simulink model "UrbanCHIL"  (Simulink 8.1)
settings: Solver=ode1  StartTime=0.0  StopTime=inf  FixedStep=Ts  MaxStep=1e-3  RelTol=1e-3
PostLoadFcn:
  | NREL_Mode=1; BANSHEE_init;
InitFcn:
  | NREL_Mode=1; BANSHEE_init;
values from neighbouring files (symbols this model uses):
  DER_REL = xlsread('DER_relay.xlsx')    [relay_settings_init.m]
  F0 = xlsread('F0_relay_banshee.xlsx')    [relay_settings_init.m]
  F2 = xlsread('F2_relay_banshee.xlsx')    [relay_settings_init.m]
  F3 = xlsread('F3_relay_banshee.xlsx')    [relay_settings_init.m]
  F4 = xlsread('F4_relay_nrel.xlsx')    [relay_settings_init.m]
  Ts = 100E-6    (= 0.0001)    [BANSHEE_init.m]    (also in Ghost_init.m)
undefined symbols (not defined in the file or in its folder): CBID, communications_lib, Feeder2_lib, Feeder3_lib, Feeder4_lib, generic_ethernet_cb, Left, relay_housing_lib, SM_UtilityService, SS_COMMUNICATION, SS_F2_RELAY_HOUSING, SS_F3_RELAY_HOUSING, SS_Feeder2, SS_Feeder3, SS_Feeder4, Stim, type, utility_service_lib, V
libraries: simulink x80, relay_modbus_lib x80, breaker_lib x46, rtio_generic_modbus x45, cables_lib x30, rtlab x22, Load_lib x21, powerlib x20, transformer_lib x19, ssn_lib x13, artemis x6, BESS_lib x4
(part 3 of 6)

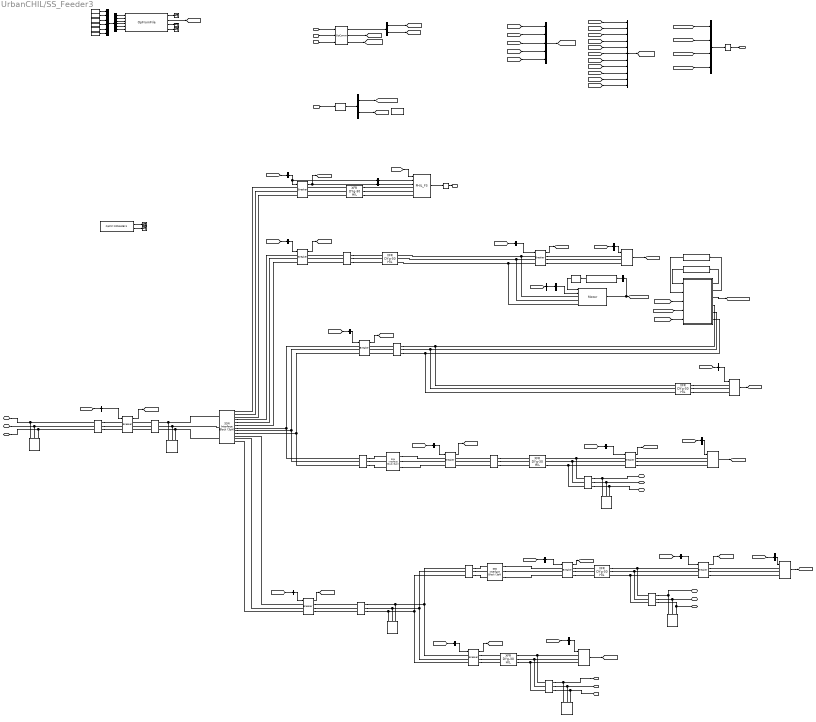
== system UrbanCHIL/SS_Feeder3 ==
  note: Signal for this Cb will come from a SEL relay
  note: connect to F2
  note: connect to F2
  note: connect to F2
  note: % Copyright (c) 2016 Massachusetts Institute of Technology
      | % Permission is hereby granted, free of charge, to any person obtaining a copy of this
      | % software and associated documentation files (the "Software"), to deal in the Software
      | % without restriction, including without limitation the rights to use, copy, modify,
      | % merge, publish, distribute, sublicense, and/or sell copies of the Software, and to
      | % permit persons to whom the Software is furnished to do so, subject to the following
      | % conditions:
      | %
      | %
      | % The above copyright notice and this permission notice shall be included in
      | % all copies or substantial portions of the Software.
      | %
      | % THE SOFTWARE IS PROVIDED "AS IS", WITHOUT WARRANTY OF ANY KIND, EXPRESS OR IMPLIED,
      | % INCLUDING BUT NOT LIMITED TO THE WARRANTIES OF MERCHANTABILITY, FITNESS FOR A
      | % PARTICULAR PURPOSE AND NONINFRINGEMENT. IN NO EVENT SHALL THE AUTHORS OR COPYRIGHT
      | % HOLDERS BE LIABLE FOR ANY CLAIM, DAMAGES OR OTHER LIABILITY, WHETHER IN AN ACTION
      | % OF CONTRACT, TORT OR OTHERWISE, ARISING FROM, OUT OF OR IN CONNECTION WITH THE
      | % SOFTWARE OR THE USE OR OTHER DEALINGS IN THE SOFTWARE.
      | %
      | %
      | %%
  note: PHIL interface
  RELAY_IN : Inport
  LOAD_IN : Inport  Port=2
  SC_CMD : Inport  Port=3
  PHIL_I : Inport  Port=4
  1000 kVA : transformer_lib/XFR DYg-30 HIL  Rating=1000  Vp=13800  Vs=480  Z=5.56  XR=5.49
  1000 kVA1 : transformer_lib/XFR DYg-30 HIL  Rating=1000  Vp=13800  Vs=480  Z=5.56  XR=5.49
  200 HP chiller compressor : Load_lib/200 HP chiller compressor
  2000 kVA : transformer_lib/XFR DYg-30 HIL  Rating=2000  Vp=13800  Vs=480  Z=5.75  XR=5.7
  2000 kVA1 : transformer_lib/XFR DYg-30 HIL  Rating=2000  Vp=13800  Vs=480  Z=5.75  XR=5.7
  2500 kVA : transformer_lib/XFR DYg-30 HIL  Rating=2500  Vp=13800  Vs=480  Z=5.75  XR=6.6
  2500 kVA1 : transformer_lib/XFR DYg-30 HIL  Rating=5000  Vp=13800  Vs=4160  Z=5.75  XR=6.6
  448 kvar inductor at 13.8kV  to cancel kvar produced by the stublines1 : powerlib/Elements/Three-Phase Parallel RLC Load  LConnTagsString=A|B|C  Configuration=Y (grounded)  NominalVoltage=13800  NominalFrequency=60  ActivePower=10e3  InductivePower=448e3  CapacitivePower=0  Measurements=None  LoadType=constant Z
  500kcmil-Mutual1 : cables_lib/500kcmil-Mutual  length=10  par_sets=1  ratio=3
  500kcmil-Mutual2 : cables_lib/500kcmil-Mutual  length=10  par_sets=1  ratio=3
  500kcmil-Mutual3 : cables_lib/500kcmil-Mutual  length=100  par_sets=1  ratio=3
  500kcmil-Mutual4 : cables_lib/500kcmil-Mutual  length=10  par_sets=1  ratio=3
  500kcmil-Mutual5 : cables_lib/500kcmil-Mutual  length=1000  par_sets=1  ratio=3
  6 kvar inductor at 480V  to cancel kvar produced by the stublines1 : powerlib/Elements/Three-Phase Parallel RLC Load  LConnTagsString=A|B|C  Configuration=Y (grounded)  NominalVoltage=480  NominalFrequency=60  ActivePower=1e3  InductivePower=6e3  CapacitivePower=0  Measurements=None  LoadType=constant Z
  6 kvar inductor at 480V  to cancel kvar produced by the stublines2 : powerlib/Elements/Three-Phase Parallel RLC Load  LConnTagsString=A|B|C  Configuration=Y (grounded)  NominalVoltage=480  NominalFrequency=60  ActivePower=1e3  InductivePower=6e3  CapacitivePower=0  Measurements=None  LoadType=constant Z
  6 kvar inductor at 480V  to cancel kvar produced by the stublines3 : powerlib/Elements/Three-Phase Parallel RLC Load  LConnTagsString=A|B|C  Configuration=Y (grounded)  NominalVoltage=480  NominalFrequency=60  ActivePower=0  InductivePower=6e3  CapacitivePower=0  Measurements=None  LoadType=constant Z
  Bus Creator2 : BusCreator
  Bus Creator3 : BusCreator  Inputs=5
  Bus Creator5 : BusCreator  Inputs=11
  Bus Selector : BusSelector  OutputSignals=motor
  Bus Selector1 : BusSelector  OutputSignals=F3_CB_4
  Bus Selector10 : BusSelector  OutputSignals=F3_CB_5
  Bus Selector11 : BusSelector  OutputSignals=P6
  Bus Selector12 : BusSelector  OutputSignals=F3_CB_9
  Bus Selector13 : BusSelector  OutputSignals=F3_CB_3
  Bus Selector14 : BusSelector  OutputSignals=F3_CB_8
  Bus Selector15 : BusSelector  OutputSignals=CHP_cmds,IO_scaling
  Bus Selector16 : BusSelector  OutputSignals=Status
  Bus Selector17 : BusSelector  OutputSignals=RPM
  Bus Selector18 : BusSelector  OutputSignals=LoadProfile,TestSeq
  Bus Selector19 : BusSelector  OutputSignals=Logic_trip
  Bus Selector2 : BusSelector  OutputSignals=C6
  Bus Selector20 : BusSelector  OutputSignals=ena2
  Bus Selector21 : BusSelector  OutputSignals=F3_PCC
  Bus Selector22 : BusSelector  OutputSignals=F3_CB_10
  Bus Selector3 : BusSelector  OutputSignals=P4
  Bus Selector4 : BusSelector  OutputSignals=I6
  Bus Selector5 : BusSelector  OutputSignals=C5
  Bus Selector6 : BusSelector  OutputSignals=F3_CB_2
  Bus Selector7 : BusSelector  OutputSignals=F3_CB_7
  Bus Selector8 : BusSelector  OutputSignals=F3_CB_6
  Bus Selector9 : BusSelector  OutputSignals=F3_CB_1
  C1 : cables_lib/500kcmil-Mutual  length=10  par_sets=1  ratio=3
  C2 : cables_lib/500kcmil-Mutual  length=10  par_sets=1  ratio=3
  C301 : cables_lib/500kcmil-Mutual  length=2500  par_sets=1  ratio=3
  C302 : cables_lib/4//0AWG-Mutual  length=2000  par_sets=1  ratio=3
  C303 : cables_lib/500kcmil-Mutual  length=2000  par_sets=1  ratio=3
  C304 : cables_lib/4//0AWG-Mutual  length=1500  par_sets=2  ratio=3
  CHP_Modbus : rtio_generic_modbus/Modbus device  conf_name=CHP_modbus.opal  conf_name_mask=CHP_modbus.xls  sample_time=Ts
  Critical_5 : Load_lib/Dynamic_Load  V=480  kVA=1000  PF=0.9  Ts=Ts
  Critical_6 : Load_lib/Dynamic_Load  V=480  kVA=800  PF=0.9  Ts=Ts
  Demux2 : Demux  Outputs=6
  F3_CB_{1..6,8..11} (10 alike) : breaker_lib/Breaker  Ts=Ts  mech_delay=cb_mech_delay
  F3_PCC : breaker_lib/Breaker  Ts=Ts  mech_delay=cb_mech_delay
  First-Order Filter : powerlib_meascontrol/Filters/First-Order Filter  FilterType=Lowpass  Tc=10e-3  Ts=Ts  Initialize=on  Vac_Init=[0, 0, 60]  Vdc_Init=0  PlotResponse=off  FreqRange="[0,  200,  1]"
  GEN2_Modbus : rtio_generic_modbus/Modbus device  conf_name=GEN2_modbus.opal  conf_name_mask=GEN2_modbus.xls  sample_time=Ts
  Goto Tag Visibility : GotoTagVisibility  GotoTag=phil_ctrl
  "Interpolation " : Constant
  Interruptible_6 : Load_lib/Dynamic_Load  V=480  kVA=600  PF=0.9  Ts=Ts
  Losses1 : powerlib/Elements/Three-Phase Parallel RLC Load  LConnTagsString=A|B|C  Configuration=Y (grounded)  NominalVoltage=13800  NominalFrequency=60  ActivePower=1e3  InductivePower=0  CapacitivePower=0  Measurements=None  LoadType=constant Z
  Losses4 : powerlib/Elements/Three-Phase Parallel RLC Load  LConnTagsString=A|B|C  Configuration=Y (grounded)  NominalVoltage=13800  NominalFrequency=60  ActivePower=1e3  InductivePower=0  CapacitivePower=0  Measurements=None  LoadType=constant Z
  Memory : Memory
  Memory1 : Memory
  Motor : Motor_InductionMachine_lib/Motor
  Mux : Mux  Inputs=6
  NGCHP_Generator : Subsystem
  OpComm1 : rtlab/OpComm  nbport=3  groupe_acq=1  subsys_rate=0  st=0  Synchronization=on  Interpolation=on  Threshold=1.0  Missed_Data=off  Sim_Time=off  Samples=off  dynSigOut=off  from_console=0  warning_done=off  writeOpCommFile=off  Offset=off
  OpComm2 : rtlab/OpComm  nbport=1  groupe_acq=1  subsys_rate=0  st=0  Synchronization=on  Interpolation=on  Threshold=1.0  Missed_Data=off  Sim_Time=off  Samples=off  dynSigOut=off  from_console=1  warning_done=off  writeOpCommFile=off  Offset=off
  OpCtrl OP5142EX1 : rtio_opalrt_op5142ex1/OpCtrl OP5142EX1  CtrlName='OP5142EX1 Ctrl'  boardid=0  BitstreamFilename=OP5142_1-EX-0000-2_1-96IO-04-01.bin  numconfig=-1  mode=Master  externalClock=off  decimRtsi=0  calibIO=off  SampleTime=0  loadinport=-1
  OpFromFile : rtlab/DataLogging/OpFromFile  filename_mode=Static (same filename all the time)  reload_mode=Next time model is paused (Real-Time)  init_file_id=0  filename=HeatLoad.mat  rtpath='./'  nrtpath='.\'  sample_time=Ts
  PHIL_F3 : PHIL_lib/PHIL_F3
  Priority_4 : Load_lib/Dynamic_Load  V=480  kVA=600  PF=0.9  Ts=Ts
  Priority_6 : Load_lib/Dynamic_Load  V=480  kVA=1000  PF=0.9  Ts=Ts
  "Repetative " : Constant
  SSN Interface Block (3ph)1 : ssn_lib/SSN Interface Block (3ph)  nb_phase=3  nb_port=2  p1_type=V-type(Left)  p2_type=V-type (Right)  p3_type=V-type(Left)  p4_type=V-type(Left)  p5_type=V-type(Left)  p6_type=V-type(Left)  p7_type=V-type(Left)  p8_type=V-type(Left)  p9_type=V-type(Left)  p10_type=V-type(Left)  p11_type=V-type(Left)  p12_type=V-type(Left)  p13_type=V-type(Left)  p14_type=V-type(Left)  p15_type=V-type(Left)  p16_type=V-type(Left)  I_port_shunt_resistance=1e9
  SSN Interface Block (3ph)2 : ssn_lib/SSN Interface Block (3ph)  nb_phase=3  nb_port=2  p1_type=V-type(Left)  p2_type=V-type (Right)  p3_type=V-type(Left)  p4_type=V-type(Left)  p5_type=V-type(Left)  p6_type=V-type(Left)  p7_type=V-type(Left)  p8_type=V-type(Left)  p9_type=V-type(Left)  p10_type=V-type(Left)  p11_type=V-type(Left)  p12_type=V-type(Left)  p13_type=V-type(Left)  p14_type=V-type(Left)  p15_type=V-type(Left)  p16_type=V-type(Left)  I_port_shunt_resistance=1e9
  SSN Interface Block (3ph)5 : ssn_lib/SSN Interface Block (3ph)  nb_phase=3  nb_port=5  p1_type=V-type(Left)  p2_type=V-type (Right)  p3_type=V-type (Right)  p4_type=V-type (Right)  p5_type=V-type (Right)  p6_type=V-type(Left)  p7_type=V-type(Left)  p8_type=V-type(Left)  p9_type=V-type(Left)  p10_type=V-type(Left)  p11_type=V-type(Left)  p12_type=V-type(Left)  p13_type=V-type(Left)  p14_type=V-type(Left)  p15_type=V-type(Left)  p16_type=V-type(Left)  I_port_shunt_resistance=1e9
  "Start_Index " : Constant
  "State " : Constant
  "Stop_Index " : Constant  Value=1800-1
  Terminator{,1..4} (5 alike) : Terminator
  "Time_Scale_Factor " : Constant
  A_CB_5 : PMIOPort  Port=1  Side=Right
  B_CB_5 : PMIOPort  Port=2  Side=Right
  C_CB_5 : PMIOPort  Port=3  Side=Right
  A_CB_6 : PMIOPort  Port=4  Side=Right
  B_CB_6 : PMIOPort  Port=5  Side=Right
  C_CB_6 : PMIOPort  Port=6  Side=Right
  A_CB_7 : PMIOPort  Port=7  Side=Right
  B_CB_7 : PMIOPort  Port=8  Side=Right
  C_CB_7 : PMIOPort  Port=9  Side=Right
  PCC_A : PMIOPort  Port=10  Side=Left
  PCC_B : PMIOPort  Port=11  Side=Left
  PCC_C : PMIOPort  Port=12  Side=Left
  DATA_OUT : Outport
  PHIL_V : Outport  Port=2
  tag scope: phil_ctrl=scoped
  wires:
  Bus Selector1/1 -> F3_CB_4/1  "<F3_CB_4>"
  LOAD_IN/1 -> OpComm1/1
  OpComm1/1 -> Bus Selector18/1
  [LOAD_IN] -> Bus Selector2/1
  [LOAD_IN] -> Bus Selector3/1
  [LOAD_IN] -> Bus Selector4/1
  [LOAD_IN] -> Bus Selector5/1
  Bus Selector2/1 -> Critical_6/1  "<C6>"
  Bus Selector3/1 -> Priority_4/1  "<P4>"
  Bus Selector4/1 -> Interruptible_6/1  "<I6>"
  Bus Selector5/1 -> Critical_5/1  "<C5>"
  Critical_6/1 -> [LOAD_C6]
  Priority_4/1 -> [LOAD_P4]
  Interruptible_6/1 -> [LOAD_I6]
  Critical_5/1 -> [LOAD_C5]
  [LOAD_C6] -> Bus Creator3/2  "F3_C6"
  [LOAD_C5] -> Bus Creator3/1  "F3_C5"
  [LOAD_I6] -> Bus Creator3/3  "F3_I6"
  [LOAD_P4] -> Bus Creator3/4  "F3_P4"
  Bus Creator3/1 -> [LOAD_DATA]  "LOAD"
  F3_CB_4/1 -> [F3_CB_4]
  F3_CB_3/1 -> [F3_CB_3]
  F3_CB_2/1 -> [F3_CB_2]
  F3_CB_6/1 -> [F3_CB_6]
  F3_CB_1/1 -> [F3_CB_1]
  F3_CB_5/1 -> [F3_CB_5]
  [F3_CB_1] -> Bus Creator5/1  "F3_CB_1"
  [F3_CB_5] -> Bus Creator5/5  "F3_CB_5"
  [F3_CB_7] -> Bus Creator5/7  "F3_CB_7"
  [F3_CB_6] -> Bus Creator5/6  "F3_CB_6"
  [F3_CB_3] -> Bus Creator5/3  "F3_CB_3"
  [F3_CB_2] -> Bus Creator5/2  "F3_CB_2"
  [F3_CB_4] -> Bus Creator5/4  "F3_CB_4"
  Bus Creator5/1 -> [CB_DATA]
  [RELAY_IN] -> Bus Selector1/1
  RELAY_IN/1 -> OpComm1/2
  OpComm1/2 -> [RELAY_IN]
  Bus Selector6/1 -> F3_CB_2/1  "<F3_CB_2>"
  [RELAY_IN] -> Bus Selector6/1
  Bus Selector7/1 -> F3_CB_11/1  "<F3_CB_7>"
  [RELAY_IN] -> Bus Selector7/1
  Bus Selector8/1 -> F3_CB_6/1  "<F3_CB_6>"
  [RELAY_IN] -> Bus Selector8/1
  Bus Selector9/1 -> F3_CB_1/1  "<F3_CB_1>"
  [RELAY_IN] -> Bus Selector9/1
  Bus Selector10/1 -> F3_CB_5/1  "<F3_CB_5>"
  [RELAY_IN] -> Bus Selector10/1
  Bus Selector13/1 -> F3_CB_3/1  "<F3_CB_3>"
  [RELAY_IN] -> Bus Selector13/1
  F3_CB_11/1 -> [F3_CB_7]
  F3_PCC/1 -> [F3_PCC]
  [F3_PCC] -> Bus Creator5/11  "F3_PCC"
  [LOAD_IN] -> Bus Selector11/1
  Bus Selector11/1 -> Priority_6/1  "<P6>"
  Priority_6/1 -> [LOAD_P6]
  [LOAD_P6] -> Bus Creator3/5  "F3_P6"
  F3_CB_9/1 -> [F3_CB_9]
  Bus Selector12/1 -> F3_CB_9/1  "<F3_CB_9>"
  [RELAY_IN] -> Bus Selector12/1
  F3_CB_8/1 -> [F3_CB_8]
  Bus Selector14/1 -> F3_CB_8/1  "<F3_CB_8>"
  [RELAY_IN] -> Bus Selector14/1
  [F3_CB_8] -> Bus Creator5/8  "F3_CB_8"
  [F3_CB_9] -> Bus Creator5/9  "F3_CB_9"
  SC_CMD/1 -> OpComm2/1
  Memory/1 -> DATA_OUT/1
  "Start_Index "/1 -> Mux/3
  "Time_Scale_Factor "/1 -> Mux/5
  "State "/1 -> Mux/1
  Demux2/1 -> OpFromFile/1
  Demux2/4 -> OpFromFile/4
  OpFromFile/2 -> [heat_load]  "Heat Load MBtu/hr"
  Demux2/5 -> OpFromFile/5
  "Repetative "/1 -> Mux/2
  Demux2/3 -> OpFromFile/3
  Demux2/6 -> OpFromFile/6
  Demux2/2 -> OpFromFile/2
  Mux/1 -> Demux2/1
  "Interpolation "/1 -> Mux/6
  "Stop_Index "/1 -> Mux/4
  OpComm2/1 -> Bus Selector15/1
  Bus Creator2/1 -> Memory/1
  [CB_DATA] -> Bus Creator2/1  "CB_DATA"
  [LOAD_DATA] -> Bus Creator2/2  "LOAD_DATA"
  [NG_CHP_DATA] -> Bus Creator2/3  "NG_CHP_DATA"
  Bus Selector17/1 -> 200 HP chiller compressor/1  "<RPM>"
  200 HP chiller compressor/1 -> First-Order Filter/1
  [TestSeq] -> Bus Selector/1
  Bus Selector/1 -> Bus Selector20/1  "<motor>"
  Bus Selector21/1 -> F3_PCC/1  "<F3_PCC>"
  [RELAY_IN] -> Bus Selector21/1
  [NGCHP_Gen] -> NGCHP_Generator/3(console)
  GEN2_Modbus/1 -> NGCHP_Generator/1(ModbusIn)
  NGCHP_Generator/1(ModbusOut) -> GEN2_Modbus/1  "Gen_meas"
  NGCHP_Generator/3(Gen_meas) -> [NG_CHP_DATA]
  [heat_load] -> NGCHP_Generator/4(Heat Load MBtu/hrs)
  NGCHP_Generator/2(ModbusOutCHP) -> CHP_Modbus/1
  CHP_Modbus/1 -> NGCHP_Generator/2(ModbusIn1)
  Bus Selector15/1 -> [NGCHP_Gen]  "<CHP_cmds>"
  [RELAY_IN] -> Bus Selector22/1
  [F3_CB_10] -> Bus Creator5/10  "F3_CB_10"
  OpComm1/3 -> [PHIL_I]
  PHIL_I/1 -> OpComm1/3
  Bus Selector18/1 -> [LOAD_IN]  "<LoadProfile>"
  Bus Selector18/2 -> [TestSeq]  "<TestSeq>"
  F3_CB_10/1 -> Bus Selector16/1, [F3_CB_10]
  Bus Selector22/1 -> Bus Selector19/1, F3_CB_10/1  "<F3_CB_10>"
  Memory1/1 -> PHIL_V/1
  Bus Selector16/1 -> PHIL_F3/3  "<Status>"
  PHIL_F3/1 -> Memory1/1
  Bus Selector19/1 -> PHIL_F3/2  "<Logic_trip>"
  [PHIL_I] -> PHIL_F3/1
  Bus Selector20/1 -> Motor/2  "<ena2>"
  Bus Selector15/2 -> [phil_ctrl]  "<IO_scaling>"
  OpFromFile/4 -> Terminator2/1
  OpFromFile/1 -> Terminator3/1
  OpFromFile/3 -> Terminator4/1
  Motor/1 -> Bus Selector17/1, [MOTOR_DATA]
  [MOTOR_DATA] -> Bus Creator2/4  "MOTOR_DATA"
  [TestSeq] -> NGCHP_Generator/5(testseq)
  First-Order Filter/1 -> Motor/1
  OpCtrl OP5142EX1/1 -> Terminator/1
  OpCtrl OP5142EX1/2 -> Terminator1/1
  connections:
  C1/LConn1 -- F3_CB_5/LConn1 -- C301/RConn1 -- Losses1/LConn3
  F3_CB_6/RConn3 -- 2000 kVA1/LConn3
  C1/LConn3 -- F3_CB_5/LConn3 -- C301/RConn3 -- Losses1/LConn1
  C304/LConn1 -- F3_CB_2/RConn1
  C302/RConn3 -- NGCHP_Generator/RConn3 -- 1000 kVA1/LConn3
  C302/LConn2 -- F3_CB_3/RConn2
  C302/RConn1 -- 1000 kVA1/LConn1 -- NGCHP_Generator/RConn1
  F3_CB_6/RConn2 -- 2000 kVA1/LConn2
  C302/RConn2 -- 1000 kVA1/LConn2 -- NGCHP_Generator/RConn2
  F3_CB_5/RConn2 -- 2000 kVA/LConn2
  C302/LConn3 -- F3_CB_3/RConn3
  C1/LConn2 -- F3_CB_5/LConn2 -- C301/RConn2 -- Losses1/LConn2
  C304/LConn2 -- F3_CB_2/RConn2
  F3_CB_6/RConn1 -- 2000 kVA1/LConn1
  C302/LConn1 -- F3_CB_3/RConn1
  F3_CB_5/RConn1 -- 2000 kVA/LConn1
  F3_CB_5/RConn3 -- 2000 kVA/LConn3
  C304/LConn3 -- F3_CB_2/RConn3
  F3_CB_11/RConn1 -- Priority_4/LConn1
  F3_CB_11/RConn3 -- Priority_4/LConn3
  F3_CB_11/RConn2 -- Priority_4/LConn2
  2000 kVA1/RConn1 -- 500kcmil-Mutual2/LConn1 -- F3_CB_8/LConn1
  500kcmil-Mutual2/LConn3 -- 2000 kVA1/RConn3 -- F3_CB_8/LConn3
  2000 kVA1/RConn2 -- 500kcmil-Mutual2/LConn2 -- F3_CB_8/LConn2
  2000 kVA/RConn1 -- 500kcmil-Mutual1/LConn1 -- Critical_5/LConn1
  2000 kVA/RConn3 -- 500kcmil-Mutual1/LConn3 -- Critical_5/LConn3
  2000 kVA/RConn2 -- 500kcmil-Mutual1/LConn2 -- Critical_5/LConn2
  Motor/LConn1 -- 2500 kVA/RConn1 -- F3_CB_9/LConn1
  Motor/LConn3 -- F3_CB_9/LConn3 -- 2500 kVA/RConn3
  Motor/LConn2 -- 2500 kVA/RConn2 -- F3_CB_9/LConn2
  C304/RConn2 -- 1000 kVA/LConn2
  C304/RConn3 -- 1000 kVA/LConn3
  C304/RConn1 -- 1000 kVA/LConn1
  500kcmil-Mutual4/LConn2 -- 1000 kVA/RConn2 -- F3_CB_11/LConn2
  500kcmil-Mutual4/LConn1 -- F3_CB_11/LConn1 -- 1000 kVA/RConn1
  F3_CB_9/RConn1 -- Priority_6/LConn1
  F3_CB_9/RConn2 -- Priority_6/LConn2
  F3_CB_9/RConn3 -- Priority_6/LConn3
  F3_CB_8/RConn1 -- Interruptible_6/LConn1
  F3_CB_8/RConn2 -- Interruptible_6/LConn2
  F3_CB_8/RConn3 -- Interruptible_6/LConn3
  SSN Interface Block (3ph)5/RConn4 -- F3_CB_4/LConn1
  SSN Interface Block (3ph)5/RConn6 -- F3_CB_4/LConn3
  SSN Interface Block (3ph)5/RConn5 -- F3_CB_4/LConn2
  C2/LConn1 -- F3_CB_3/LConn1 -- SSN Interface Block (3ph)5/RConn7
  C2/LConn3 -- F3_CB_3/LConn3 -- SSN Interface Block (3ph)5/RConn9
  C2/LConn2 -- F3_CB_3/LConn2 -- SSN Interface Block (3ph)5/RConn8
  C303/LConn1 -- F3_CB_4/RConn1
  C303/LConn2 -- F3_CB_4/RConn2
  C303/LConn3 -- F3_CB_4/RConn3
  C303/RConn2 -- 2500 kVA/LConn2
  C303/RConn3 -- 2500 kVA/LConn3
  C303/RConn1 -- 2500 kVA/LConn1
  1000 kVA1/RConn1 -- Critical_6/LConn1
  1000 kVA1/RConn2 -- Critical_6/LConn2
  1000 kVA1/RConn3 -- Critical_6/LConn3
  6 kvar inductor at 480V  to cancel kvar produced by the stublines3/LConn2 -- 500kcmil-Mutual1/RConn2 -- B_CB_5/RConn1
  A_CB_5/RConn1 -- 500kcmil-Mutual1/RConn1 -- 6 kvar inductor at 480V  to cancel kvar produced by the stublines3/LConn1
  6 kvar inductor at 480V  to cancel kvar produced by the stublines3/LConn3 -- 500kcmil-Mutual1/RConn3 -- C_CB_5/RConn1
  6 kvar inductor at 480V  to cancel kvar produced by the stublines2/LConn2 -- 500kcmil-Mutual2/RConn2 -- B_CB_6/RConn1
  6 kvar inductor at 480V  to cancel kvar produced by the stublines2/LConn3 -- 500kcmil-Mutual2/RConn3 -- C_CB_6/RConn1
  6 kvar inductor at 480V  to cancel kvar produced by the stublines2/LConn1 -- A_CB_6/RConn1 -- 500kcmil-Mutual2/RConn1
  6 kvar inductor at 480V  to cancel kvar produced by the stublines1/LConn2 -- 500kcmil-Mutual4/RConn2 -- B_CB_7/RConn1
  6 kvar inductor at 480V  to cancel kvar produced by the stublines1/LConn3 -- 500kcmil-Mutual4/RConn3 -- C_CB_7/RConn1
  6 kvar inductor at 480V  to cancel kvar produced by the stublines1/LConn1 -- 500kcmil-Mutual4/RConn1 -- A_CB_7/RConn1
  500kcmil-Mutual3/LConn3 -- F3_PCC/RConn3
  500kcmil-Mutual3/LConn1 -- F3_PCC/RConn1
  500kcmil-Mutual3/LConn2 -- F3_PCC/RConn2
  500kcmil-Mutual5/RConn1 -- F3_PCC/LConn1
  500kcmil-Mutual5/RConn2 -- F3_PCC/LConn2
  500kcmil-Mutual5/RConn3 -- F3_PCC/LConn3
  500kcmil-Mutual4/LConn3 -- 1000 kVA/RConn3 -- F3_CB_11/LConn3
  C1/RConn2 -- SSN Interface Block (3ph)1/LConn2
  C1/RConn3 -- SSN Interface Block (3ph)1/LConn3
  C1/RConn1 -- SSN Interface Block (3ph)1/LConn1
  500kcmil-Mutual3/RConn1 -- SSN Interface Block (3ph)5/LConn1 -- Losses4/LConn1
  500kcmil-Mutual3/RConn2 -- SSN Interface Block (3ph)5/LConn2 -- Losses4/LConn2
  500kcmil-Mutual3/RConn3 -- SSN Interface Block (3ph)5/LConn3 -- Losses4/LConn3
  PCC_A/RConn1 -- 500kcmil-Mutual5/LConn1 -- 448 kvar inductor at 13.8kV  to cancel kvar produced by the stublines1/LConn1
  PCC_B/RConn1 -- 448 kvar inductor at 13.8kV  to cancel kvar produced by the stublines1/LConn2 -- 500kcmil-Mutual5/LConn2
  PCC_C/RConn1 -- 448 kvar inductor at 13.8kV  to cancel kvar produced by the stublines1/LConn3 -- 500kcmil-Mutual5/LConn3
  SSN Interface Block (3ph)2/RConn3 -- F3_CB_2/LConn3
  SSN Interface Block (3ph)2/RConn2 -- F3_CB_2/LConn2
  SSN Interface Block (3ph)2/RConn1 -- F3_CB_2/LConn1
  C2/RConn2 -- SSN Interface Block (3ph)2/LConn2
  C2/RConn1 -- SSN Interface Block (3ph)2/LConn1
  C2/RConn3 -- SSN Interface Block (3ph)2/LConn3
  F3_CB_1/LConn2 -- SSN Interface Block (3ph)5/RConn11
  F3_CB_1/LConn1 -- SSN Interface Block (3ph)5/RConn10
  F3_CB_1/LConn3 -- SSN Interface Block (3ph)5/RConn12
  SSN Interface Block (3ph)1/RConn1 -- F3_CB_6/LConn1
  SSN Interface Block (3ph)1/RConn2 -- F3_CB_6/LConn2
  SSN Interface Block (3ph)1/RConn3 -- F3_CB_6/LConn3
  F3_CB_1/RConn1 -- C301/LConn1
  F3_CB_1/RConn2 -- C301/LConn2
  F3_CB_1/RConn3 -- C301/LConn3
  F3_CB_10/LConn3 -- SSN Interface Block (3ph)5/RConn3
  F3_CB_10/LConn2 -- SSN Interface Block (3ph)5/RConn2
  F3_CB_10/LConn1 -- SSN Interface Block (3ph)5/RConn1
  2500 kVA1/LConn2 -- F3_CB_10/RConn2
  2500 kVA1/LConn1 -- F3_CB_10/RConn1
  2500 kVA1/LConn3 -- F3_CB_10/RConn3
  2500 kVA1/RConn3 -- PHIL_F3/LConn3
  2500 kVA1/RConn2 -- PHIL_F3/LConn2
  2500 kVA1/RConn1 -- PHIL_F3/LConn1

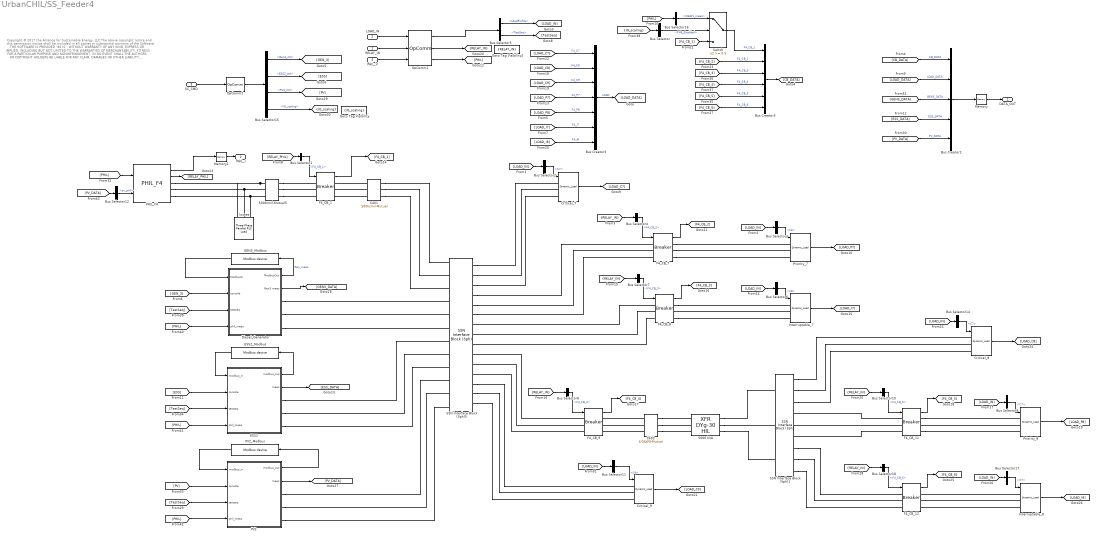
== system UrbanCHIL/SS_Feeder4 ==
  note: Copyright © 2017 the Alliance for Sustainable Energy, LLC
      |
      | The above copyright notice and this permission notice shall be included in all copies or substantial portions of the Software.
      |
      | THE SOFTWARE IS PROVIDED "AS IS", WITHOUT WARRANTY OF ANY KIND, EXPRESS OR IMPLIED, INCLUDING
      | BUT NOT LIMITED TO THE WARRANTIES OF MERCHANTABILITY, FITNESS FOR A PARTICULAR PURPOSE AND
      | NONINFRINGEMENT. IN NO EVENT SHALL THE AUTHORS OR COPYRIGHT HOLDERS BE LIABLE FOR ANY CLAIM,
      |  DAMAGES OR OTHER LIABILITY, WHETHER IN AN ACTION OF CONTRACT, TORT OR OTHERWISE, ARISING FROM,
      | OUT OF OR IN CONNECTION WITH THE SOFTWARE OR THE USE OR OTHER DEALINGS IN THE SOFTWARE
  RELAY_IN : Inport
  LOAD_IN : Inport  Port=2
  SC_CMD : Inport  Port=3
  PHIL_V : Inport  Port=4
  5000 kVA : transformer_lib/XFR DYg-30 HIL  Rating=50  Vp=480  Vs=208  Z=5.75  XR=4.7
  500kcmil-Mutual5 : cables_lib/500kcmil-Mutual  length=1000  par_sets=1  ratio=3
  Bus Creator2 : BusCreator  Inputs=5
  Bus Creator3 : BusCreator  Inputs=7
  Bus Creator5 : BusCreator  Inputs=6
  Bus Selector : BusSelector  OutputSignals=PHIL_Enabled
  Bus Selector1 : BusSelector  OutputSignals=F4_CB_1
  Bus Selector10 : BusSelector  OutputSignals=F4_CB_5
  Bus Selector11 : BusSelector  OutputSignals=C9
  Bus Selector12 : BusSelector  OutputSignals=pv_phil
  Bus Selector{2,9,14,17} (4 alike) : BusSelector  OutputSignals=C7
  Bus Selector15 : BusSelector  OutputSignals=Gen3_ctrl,ESS2_ctrl,PV2_ctrl,IO_scaling
  Bus Selector16 : BusSelector  OutputSignals=CB401_meas
  Bus Selector18 : BusSelector  OutputSignals=F4_CB_6
  Bus Selector3 : BusSelector  OutputSignals=C8
  Bus Selector4 : BusSelector  OutputSignals=F4_CB_2
  Bus Selector5 : BusSelector  OutputSignals=LoadProfile,TestSeq
  Bus Selector6 : BusSelector  OutputSignals=C8
  Bus Selector7 : BusSelector  OutputSignals=F4_CB_3
  Bus Selector8 : BusSelector  OutputSignals=F4_CB_4
  C401 : cables_lib/500kcmil-Mutual  length=2000  par_sets=1  ratio=3
  C403 : cables_lib/4//0AWG-Mutual  length=2000  par_sets=1  ratio=3
  Critical_7 : Load_lib/Dynamic_Load  V=480  kVA=25  PF=0.9  Ts=Ts
  Critical_8 : Load_lib/Dynamic_Load  V=208  kVA=20  PF=0.9  Ts=Ts
  Critical_9 : Load_lib/Dynamic_Load  V=480  kVA=3  PF=0.9  Ts=Ts
  Diesel_Generator : Subsystem
  ESS2 : Subsystem
  ESS2_Modbus : rtio_generic_modbus/Modbus device  conf_name=ESS2_modbus.opal  conf_name_mask=ESS2_modbus.xls  sample_time=Ts
  F4_CB_{1,7..9,11..12} (6 alike) : breaker_lib/Breaker  Ts=Ts  mech_delay=cb_mech_delay
  GEN3_Modbus : rtio_generic_modbus/Modbus device  conf_name=GEN3_modbus.opal  conf_name_mask=GEN3_modbus.xls  sample_time=Ts
  Goto Tag Visibility : GotoTagVisibility  GotoTag=IO_scaling
  Goto Tag Visibility2 : GotoTagVisibility  GotoTag=RELAY_IN
  Interruptable_7 : Load_lib/Dynamic_Load  V=480  kVA=30  PF=0.9  Ts=Ts
  Interruptable_8 : Load_lib/Dynamic_Load  V=208  kVA=20  PF=0.9  Ts=Ts
  Memory : Memory
  Memory1 : Memory
  OpComm1 : rtlab/OpComm  nbport=3  groupe_acq=1  subsys_rate=0  st=0  Synchronization=on  Interpolation=on  Threshold=1.0  Missed_Data=off  Sim_Time=off  Samples=off  dynSigOut=off  from_console=0  warning_done=off  writeOpCommFile=off  Offset=off
  OpComm2 : rtlab/OpComm  nbport=1  groupe_acq=1  subsys_rate=0  st=0  Synchronization=on  Interpolation=on  Threshold=1.0  Missed_Data=off  Sim_Time=off  Samples=off  dynSigOut=off  from_console=1  warning_done=off  writeOpCommFile=off  Offset=off
  PHIL_F4 : PHIL_lib/PHIL_F4
  PV2 : Subsystem
  PV2_Modbus : rtio_generic_modbus/Modbus device  conf_name=PV2_modbus.opal  conf_name_mask=PV2_modbus.xls  sample_time=Ts
  Priority_7 : Load_lib/Dynamic_Load  V=480  kVA=10  PF=0.9  Ts=Ts
  Priority_8 : Load_lib/Dynamic_Load  V=208  kVA=10  PF=0.9  Ts=Ts
  SSN Interface Block (3ph)1 : ssn_lib/SSN Interface Block (3ph)  nb_phase=3  nb_port=4  p1_type=V-type(Left)  p2_type=V-type (Right)  p3_type=V-type (Right)  p4_type=V-type (Right)  p5_type=V-type (Right)  p6_type=V-type (Right)  p7_type=V-type (Right)  p8_type=V-type(Left)  p9_type=V-type(Left)  p10_type=V-type(Left)  p11_type=V-type(Left)  p12_type=V-type(Left)  p13_type=V-type(Left)  p14_type=V-type(Left)  p15_type=V-type(Left)  p16_type=V-type(Left)  I_port_shunt_resistance=1e9
  SSN Interface Block (3ph)5 : ssn_lib/SSN Interface Block (3ph)  nb_phase=3  nb_port=9  p1_type=V-type(Left)  p2_type=V-type (Right)  p3_type=V-type (Right)  p4_type=V-type (Right)  p5_type=V-type (Right)  p6_type=V-type (Right)  p7_type=V-type(Left)  p8_type=V-type(Left)  p9_type=V-type(Left)  p10_type=V-type(Left)  p11_type=V-type(Left)  p12_type=V-type(Left)  p13_type=V-type(Left)  p14_type=V-type(Left)  p15_type=V-type(Left)  p16_type=V-type(Left)  I_port_shunt_resistance=1e9
  Switch : Switch  Threshold=0.5
  losses : powerlib/Elements/Three-Phase Parallel RLC Load  LConnTagsString=A|B|C  Configuration=Y (grounded)  NominalVoltage=480  NominalFrequency=60  ActivePower=1e3  InductivePower=1e3  CapacitivePower=0  Measurements=None  LoadType=constant Z
  DATA_OUT : Outport
  PHIL_I : Outport  Port=2
  tag scope: IO_scaling=scoped, RELAY_IN=scoped
  wires:
  Bus Selector15/1 -> [GEN_3]  "<Gen3_ctrl>"
  [GEN3_DATA] -> Bus Creator2/3  "GEN3_DATA"
  [LOAD_DATA] -> Bus Creator2/2  "LOAD_DATA"
  [CB_DATA] -> Bus Creator2/1  "CB_DATA"
  Bus Creator2/1 -> Memory/1
  OpComm2/1 -> Bus Selector15/1
  Memory/1 -> DATA_OUT/1
  SC_CMD/1 -> OpComm2/1
  F4_CB_1/1 -> [F4_CB_1]
  OpComm1/2 -> [RELAY_IN]
  RELAY_IN/1 -> OpComm1/2
  Bus Creator5/1 -> [CB_DATA]
  [F4_CB_4] -> Bus Creator5/4  "F4_CB_4"
  [F4_CB_2] -> Bus Creator5/2  "F4_CB_2"
  [F4_CB_3] -> Bus Creator5/3  "F4_CB_3"
  [F4_CB_6] -> Bus Creator5/6  "F4_CB_6"
  [F4_CB_5] -> Bus Creator5/5  "F4_CB_5"
  Switch/1 -> Bus Creator5/1  "F4_CB_1"
  Bus Creator3/1 -> [LOAD_DATA]  "LOAD"
  [LOAD_C9] -> Bus Creator3/3  "F4_C9"
  [LOAD_C7] -> Bus Creator3/1  "F4_C7"
  [LOAD_C8] -> Bus Creator3/2  "F4_C8"
  LOAD_IN/1 -> OpComm1/1
  Critical_9/1 -> [LOAD_C9]
  Bus Selector11/1 -> Critical_9/1  "<C9>"
  [LOAD_IN] -> Bus Selector11/1
  Critical_7/1 -> [LOAD_C7]
  Bus Selector2/1 -> Critical_7/1  "<C7>"
  [LOAD_IN] -> Bus Selector2/1
  Priority_7/1 -> [LOAD_P7]
  Bus Selector3/1 -> Priority_7/1  "<C8>"
  [LOAD_IN] -> Bus Selector3/1
  [RELAY_IN] -> Bus Selector4/1
  Bus Selector4/1 -> F4_CB_7/1  "<F4_CB_2>"
  F4_CB_7/1 -> [F4_CB_2]
  [GEN_3] -> Diesel_Generator/2(console)
  Bus Selector15/2 -> [ESS]  "<ESS2_ctrl>"
  [ESS_DATA] -> Bus Creator2/4  "ESS_DATA"
  [ESS] -> ESS2/2(console)
  Interruptable_7/1 -> [LOAD_I7]
  Bus Selector6/1 -> Interruptable_7/1  "<C8>"
  [LOAD_IN] -> Bus Selector6/1
  [RELAY_IN] -> Bus Selector7/1
  Bus Selector7/1 -> F4_CB_8/1  "<F4_CB_3>"
  F4_CB_8/1 -> [F4_CB_3]
  [RELAY_IN] -> Bus Selector8/1
  Bus Selector8/1 -> F4_CB_9/1  "<F4_CB_4>"
  F4_CB_9/1 -> [F4_CB_4]
  Priority_8/1 -> [LOAD_P8]
  Bus Selector9/1 -> Priority_8/1  "<C7>"
  [LOAD_IN] -> Bus Selector9/1
  [RELAY_IN] -> Bus Selector10/1
  Bus Selector10/1 -> F4_CB_11/1  "<F4_CB_5>"
  F4_CB_11/1 -> [F4_CB_5]
  Critical_8/1 -> [LOAD_C8]
  Bus Selector14/1 -> Critical_8/1  "<C7>"
  [LOAD_IN] -> Bus Selector14/1
  Interruptable_8/1 -> [LOAD_I8]
  Bus Selector17/1 -> Interruptable_8/1  "<C7>"
  [LOAD_IN] -> Bus Selector17/1
  [RELAY_IN] -> Bus Selector18/1
  Bus Selector18/1 -> F4_CB_12/1  "<F4_CB_6>"
  F4_CB_12/1 -> [F4_CB_6]
  [PV_DATA] -> Bus Creator2/5  "PV_DATA"
  Bus Selector15/3 -> [PV]  "<PV2_ctrl>"
  PV2_Modbus/1 -> PV2/1(modbus_in)
  PV2/1(modbus_out) -> PV2_Modbus/1
  PV2/2(meas) -> [PV_DATA]
  ESS2/2(meas) -> [ESS_DATA]
  ESS2/1(modbus_out) -> ESS2_Modbus/1
  ESS2_Modbus/1 -> ESS2/1(modbus_in)
  GEN3_Modbus/1 -> Diesel_Generator/1(ModbusIn)
  Diesel_Generator/1(ModbusOut) -> GEN3_Modbus/1  "Gen_meas"
  Diesel_Generator/2(Gen3 meas) -> [GEN3_DATA]
  [LOAD_I7] -> Bus Creator3/6  "F4_I7"
  [LOAD_P7] -> Bus Creator3/4  "F4_P7"
  [LOAD_P8] -> Bus Creator3/5  "F4_P8"
  [LOAD_I8] -> Bus Creator3/7  "F4_I8"
  Memory1/1 -> PHIL_I/1
  PHIL_V/1 -> OpComm1/3
  OpComm1/3 -> [PHIL]
  OpComm1/1 -> Bus Selector5/1
  Bus Selector5/1 -> [LOAD_IN]  "<LoadProfile>"
  Bus Selector5/2 -> [TestSeq]  "<TestSeq>"
  Bus Selector15/4 -> [IO_scaling]  "<IO_scaling>"
  PHIL_F4/1 -> Memory1/1
  PHIL_F4/2 -> [RELAY_PHIL]
  [RELAY_PHIL] -> Bus Selector1/1
  Bus Selector1/1 -> F4_CB_1/1  "<F4_CB_1>"
  Bus Selector16/1 -> Switch/1  "<CB401_meas>"
  [IO_scaling] -> Bus Selector/1
  Bus Selector/1 -> Switch/2  "<PHIL_Enabled>"
  [PHIL] -> Bus Selector16/1
  [F4_CB_1] -> Switch/3
  [PHIL] -> PHIL_F4/1
  [TestSeq] -> PV2/3(testseq)
  [PV] -> PV2/2(console)
  [TestSeq] -> ESS2/3(testseq)
  [TestSeq] -> Diesel_Generator/3(testseq)
  [PHIL] -> Diesel_Generator/4(phil_meas)
  [PHIL] -> ESS2/4(phil_meas)
  [PHIL] -> PV2/4(phil_meas)
  [PV_DATA] -> Bus Selector12/1
  Bus Selector12/1 -> PHIL_F4/2  "<pv_phil>"
  connections:
  losses/LConn3 -- PHIL_F4/RConn3 -- 500kcmil-Mutual5/LConn3
  losses/LConn2 -- PHIL_F4/RConn2 -- 500kcmil-Mutual5/LConn2
  500kcmil-Mutual5/LConn1 -- PHIL_F4/RConn1 -- losses/LConn1
  C401/RConn3 -- SSN Interface Block (3ph)5/LConn3
  C401/RConn2 -- SSN Interface Block (3ph)5/LConn2
  C401/RConn1 -- SSN Interface Block (3ph)5/LConn1
  500kcmil-Mutual5/RConn3 -- F4_CB_1/LConn3
  500kcmil-Mutual5/RConn2 -- F4_CB_1/LConn2
  500kcmil-Mutual5/RConn1 -- F4_CB_1/LConn1
  C401/LConn2 -- F4_CB_1/RConn2
  C401/LConn1 -- F4_CB_1/RConn1
  C401/LConn3 -- F4_CB_1/RConn3
  F4_CB_7/RConn2 -- Priority_7/LConn2
  F4_CB_7/RConn3 -- Priority_7/LConn3
  F4_CB_7/RConn1 -- Priority_7/LConn1
  SSN Interface Block (3ph)5/RConn6 -- F4_CB_7/LConn3
  SSN Interface Block (3ph)5/RConn5 -- F4_CB_7/LConn2
  SSN Interface Block (3ph)5/RConn4 -- F4_CB_7/LConn1
  SSN Interface Block (3ph)5/RConn1 -- Critical_7/LConn1
  SSN Interface Block (3ph)5/RConn3 -- Critical_7/LConn3
  SSN Interface Block (3ph)5/RConn2 -- Critical_7/LConn2
  F4_CB_8/LConn1 -- SSN Interface Block (3ph)5/RConn7
  F4_CB_8/LConn2 -- SSN Interface Block (3ph)5/RConn8
  F4_CB_8/LConn3 -- SSN Interface Block (3ph)5/RConn9
  F4_CB_8/RConn1 -- Interruptable_7/LConn1
  F4_CB_8/RConn3 -- Interruptable_7/LConn3
  Interruptable_7/LConn2 -- F4_CB_8/RConn2
  C403/LConn1 -- F4_CB_9/RConn1
  C403/LConn3 -- F4_CB_9/RConn3
  C403/LConn2 -- F4_CB_9/RConn2
  F4_CB_9/LConn3 -- SSN Interface Block (3ph)5/RConn12
  F4_CB_9/LConn1 -- SSN Interface Block (3ph)5/RConn10
  F4_CB_9/LConn2 -- SSN Interface Block (3ph)5/RConn11
  C403/RConn2 -- 5000 kVA/LConn2
  C403/RConn1 -- 5000 kVA/LConn1
  C403/RConn3 -- 5000 kVA/LConn3
  5000 kVA/RConn2 -- SSN Interface Block (3ph)1/LConn2
  5000 kVA/RConn3 -- SSN Interface Block (3ph)1/LConn3
  5000 kVA/RConn1 -- SSN Interface Block (3ph)1/LConn1
  Priority_8/LConn2 -- F4_CB_11/RConn2
  F4_CB_11/RConn1 -- Priority_8/LConn1
  F4_CB_11/RConn3 -- Priority_8/LConn3
  Interruptable_8/LConn1 -- F4_CB_12/RConn1
  Interruptable_8/LConn3 -- F4_CB_12/RConn3
  F4_CB_12/RConn2 -- Interruptable_8/LConn2
  SSN Interface Block (3ph)1/RConn3 -- Critical_8/LConn3
  SSN Interface Block (3ph)1/RConn2 -- Critical_8/LConn2
  SSN Interface Block (3ph)1/RConn1 -- Critical_8/LConn1
  F4_CB_11/LConn3 -- SSN Interface Block (3ph)1/RConn6
  F4_CB_11/LConn2 -- SSN Interface Block (3ph)1/RConn5
  F4_CB_11/LConn1 -- SSN Interface Block (3ph)1/RConn4
  SSN Interface Block (3ph)1/RConn9 -- F4_CB_12/LConn3
  SSN Interface Block (3ph)1/RConn8 -- F4_CB_12/LConn2
  SSN Interface Block (3ph)1/RConn7 -- F4_CB_12/LConn1
  Diesel_Generator/RConn1 -- SSN Interface Block (3ph)5/LConn4
  Diesel_Generator/RConn2 -- SSN Interface Block (3ph)5/LConn5
  Diesel_Generator/RConn3 -- SSN Interface Block (3ph)5/LConn6
  ESS2/RConn3 -- SSN Interface Block (3ph)5/LConn9
  ESS2/RConn1 -- SSN Interface Block (3ph)5/LConn7
  ESS2/RConn2 -- SSN Interface Block (3ph)5/LConn8
  PV2/RConn1 -- SSN Interface Block (3ph)5/LConn10
  PV2/RConn2 -- SSN Interface Block (3ph)5/LConn11
  PV2/RConn3 -- SSN Interface Block (3ph)5/LConn12
  SSN Interface Block (3ph)5/RConn15 -- Critical_9/LConn3
  SSN Interface Block (3ph)5/RConn14 -- Critical_9/LConn2
  SSN Interface Block (3ph)5/RConn13 -- Critical_9/LConn1

== system UrbanCHIL/SC_ctrl/CB_modbus_mock ==
  note: Should be from pattern generator
  Bus Creator1 : BusCreator  Inputs=7
  Enabled : Constant
  F1 : Subsystem
  F2 : Subsystem
  F3 : Subsystem
  F4 : Subsystem
  Manual Switch{,1..3} (4 alike) : ManualSwitch
  Manual Switch4 : ManualSwitch  CurrentSetting=0
  NO FAULT : Constant  Value=0
  NO FAULT2 : Constant  Value=0
  NO FAULT3 : Constant  Value=0
  Pulse Generator : DiscretePulseGenerator  SampleTime=[Stim.Ts Ts]
  RST : Constant
  Rate Transition : RateTransition  Deterministic=off
  setting #1 : Constant  Value=0
  setting #2 : Constant
  Out1 : Outport
  wires:
  Bus Creator1/1 -> Rate Transition/1
  F4/1(Out1) -> Bus Creator1/4  "F4"
  F3/1(Out1) -> Bus Creator1/3  "F3"
  F2/1(Out1) -> Bus Creator1/2  "F2"
  F1/1(Out1) -> Bus Creator1/1  "F1"
  Manual Switch/1 -> Bus Creator1/5  "ResetAll"
  Manual Switch1/1 -> Manual Switch/2
  Pulse Generator/1 -> Manual Switch/1
  NO FAULT/1 -> Manual Switch1/1
  RST/1 -> Manual Switch1/2  "record_rms_signals"
  Manual Switch3/1 -> Manual Switch2/2
  NO FAULT2/1 -> Manual Switch2/1
  setting #1/1 -> Manual Switch3/1
  setting #2/1 -> Manual Switch3/2  "record_rms_signals"
  Manual Switch2/1 -> Bus Creator1/6  "GroupSel"
  Manual Switch4/1 -> Bus Creator1/7  "MockEna"
  NO FAULT3/1 -> Manual Switch4/1
  Enabled/1 -> Manual Switch4/2  "record_rms_signals"
  Rate Transition/1 -> Out1/1

== system UrbanCHIL/SC_ctrl/Gen1_Modbus_Stimuli2 ==
  note: Use Modbus from
      | Console
  note: Use Modbus TCP
  Bus Creator1 : BusCreator  Inputs=2
  Bus Creator12 : BusCreator  Inputs=8
  Fcmd pu : Constant  Value=1.003
  Gain3 : Gain  Gain=4000
  Gain4 : Gain  Gain=4000
  Gain5 : Gain  Gain=13800
  Gain6 : Gain  Gain=6000
  Manual Switch2 : ManualSwitch
  Manual Switch3 : ManualSwitch
  Manual Switch4 : ManualSwitch
  PCmd1 : Constant  Value=300
  PCmd2 : Constant  Value=300
  PCmd3 : Constant  Value=0
  PCmd4 : Constant  Value=0
  PCmd5 : Constant  Value=12
  PCmd6 : Constant  Value=0
  PCmd7 : Constant
  PCmd8 : Constant  Value=11
  Pfactor : Gain  Gain=.9
  Qfactor : Gain  Gain=.43
  Rate Transition1 : RateTransition  Deterministic=off
  S Profile3 : simulink/Sources/Repeating Sequence Stair  OutValues=Stim.Gen3.s  tsamp=[Stim.Ts Ts]  OutMin=[]  OutMax=[]  OutDataTypeStr=Inherit: Inherit via back propagation  OutDataType=fixdt(0,8)  ConRadixGroup=Best Precision: Vector-wise  OutScaling=2^-12
  Vcmd pu : Constant
  MbCtrl : Outport
  wires:
  S Profile3/1 -> Pfactor/1, Qfactor/1  "P"
  Qfactor/1 -> Manual Switch3/1  "Q"
  Vcmd pu/1 -> Gain5/1  "V"
  Fcmd pu/1 -> Gain6/1  "F"
  Pfactor/1 -> Manual Switch2/1  "P"
  Manual Switch2/1 -> Gain3/1
  Bus Creator12/1 -> Bus Creator1/1  "ModbusFromSC"
  Manual Switch3/1 -> Gain4/1
  PCmd4/1 -> Manual Switch3/2
  PCmd3/1 -> Manual Switch2/2
  PCmd1/1 -> Bus Creator12/6
  PCmd2/1 -> Bus Creator12/7
  PCmd5/1 -> Bus Creator12/8
  Bus Creator1/1 -> Rate Transition1/1
  Manual Switch4/1 -> Bus Creator1/2  "ModbusEnable"
  PCmd6/1 -> Manual Switch4/1
  PCmd7/1 -> Manual Switch4/2
  Gain3/1 -> Bus Creator12/2  "PCmd"
  Gain4/1 -> Bus Creator12/3  "QCmd"
  Gain5/1 -> Bus Creator12/4  "VoltCmd"
  Gain6/1 -> Bus Creator12/5  "FreqCmd"
  Rate Transition1/1 -> MbCtrl/1
  PCmd8/1 -> Bus Creator12/1  "Ctrl"

== system UrbanCHIL/SC_ctrl/Gen2_NGCHP_Modbus_Stimuli ==
  note: Use Modbus TCP
  note: Use Modbus from
      | Console
  note: Enable
  note: Reset
  MainsCon : Inport
  Bus Creator1 : BusCreator  Inputs=3
  Bus Creator10 : BusCreator  Inputs=3
  Bus Creator12 : BusCreator  Inputs=8
  CHP Enable/Disable : ManualSwitch  CurrentSetting=0
  CHP Reset : ManualSwitch  CurrentSetting=0
  CHP TempSetPoint : Constant  Value=20.05
  Constant3 : Constant  Value=0
  Constant4 : Constant
  Fcmd pu : Constant  Value=1.003
  Gain1 : Gain  Gain=2  OutDataTypeStr=double
  Gain2 : Gain
  Gain3 : Gain  Gain=3500
  Gain4 : Gain  Gain=3500
  Gain5 : Gain  Gain=13800
  Gain6 : Gain  Gain=6000
  Gain7 : Gain  Gain=8
  Logical Operator : Logic  Operator=NOT  AllPortsSameDT=off  OutDataTypeStr=boolean
  Manual Switch1 : ManualSwitch  CurrentSetting=0
  Manual Switch2 : ManualSwitch
  Manual Switch3 : ManualSwitch
  Manual Switch4 : ManualSwitch
  PCmd1 : Constant  Value=300
  PCmd2 : Constant  Value=300
  PCmd3 : Constant  Value=0
  PCmd4 : Constant  Value=0
  PCmd5 : Constant  Value=14
  PCmd6 : Constant  Value=0
  PCmd7 : Constant
  PCmd8 : Constant  Value=11
  Pfactor : Gain  Gain=.9
  Qfactor : Gain  Gain=.43
  Rate Transition : RateTransition  Deterministic=off
  Rate Transition1 : RateTransition  Deterministic=off
  S Profile1 : simulink/Sources/Repeating Sequence Stair  OutValues=Stim.Gen3.Ena  tsamp=[Stim.Ts Ts]  OutMin=[]  OutMax=[]  OutDataTypeStr=Inherit: Inherit via back propagation  OutDataType=fixdt(0,8)  ConRadixGroup=Best Precision: Vector-wise  OutScaling=2^-12
  S Profile2 : simulink/Sources/Repeating Sequence Stair  OutValues=Stim.Gen3.Run  tsamp=[Stim.Ts Ts]  OutMin=[]  OutMax=[]  OutDataTypeStr=Inherit: Inherit via back propagation  OutDataType=fixdt(0,8)  ConRadixGroup=Best Precision: Vector-wise  OutScaling=2^-12
  S Profile3 : simulink/Sources/Repeating Sequence Stair  OutValues=Stim.Gen3.s  tsamp=[Stim.Ts Ts]  OutMin=[]  OutMax=[]  OutDataTypeStr=Inherit: Inherit via back propagation  OutDataType=fixdt(0,8)  ConRadixGroup=Best Precision: Vector-wise  OutScaling=2^-12
  Sum : Sum  Inputs=+++
  Vcmd pu : Constant
  MbCtrl : Outport
  wires:
  Rate Transition/1 -> Logical Operator/1
  Logical Operator/1 -> Gain1/1  "VF_control"
  MainsCon/1 -> Rate Transition/1
  Gain7/1 -> Sum/3
  S Profile2/1 -> Gain7/1  "Run"
  Gain6/1 -> Bus Creator12/5  "FreqCmd"
  Gain5/1 -> Bus Creator12/4  "VoltCmd"
  Gain4/1 -> Bus Creator12/3  "QCmd"
  Gain3/1 -> Bus Creator12/2  "PCmd"
  PCmd7/1 -> Manual Switch4/2
  PCmd6/1 -> Manual Switch4/1
  Manual Switch4/1 -> Bus Creator1/2  "ModbusEnable"
  Bus Creator1/1 -> Rate Transition1/1
  PCmd5/1 -> Bus Creator12/8
  PCmd2/1 -> Bus Creator12/7
  PCmd1/1 -> Bus Creator12/6
  Sum/1 -> Manual Switch1/1
  Gain1/1 -> Sum/2
  Gain2/1 -> Sum/1
  PCmd3/1 -> Manual Switch2/2
  PCmd4/1 -> Manual Switch3/2
  Manual Switch3/1 -> Gain4/1
  Bus Creator12/1 -> Bus Creator1/1  "ModbusFromSC"
  Manual Switch2/1 -> Gain3/1
  S Profile1/1 -> Gain2/1  "Enable"
  Pfactor/1 -> Manual Switch2/1  "P"
  Fcmd pu/1 -> Gain6/1  "F"
  Vcmd pu/1 -> Gain5/1  "V"
  Qfactor/1 -> Manual Switch3/1  "Q"
  S Profile3/1 -> Qfactor/1, Pfactor/1  "P"
  Bus Creator10/1 -> Bus Creator1/3  "CHP_SIM_Cmds"
  CHP Reset/1 -> Bus Creator10/3  "CHP Reset"
  CHP TempSetPoint/1 -> Bus Creator10/2  "CHP TempSetPoint"
  CHP Enable/Disable/1 -> Bus Creator10/1  "CHP Enable/Disable"
  Constant4/1 -> CHP Enable/Disable/1, CHP Reset/1
  Constant3/1 -> CHP Enable/Disable/2, CHP Reset/2
  Rate Transition1/1 -> MbCtrl/1
  PCmd8/1 -> Manual Switch1/2
  Manual Switch1/1 -> Bus Creator12/1  "Ctrl"

== system UrbanCHIL/SC_ctrl/Gen3_Modbus_Stimuli1 ==
  note: Use Modbus TCP
  note: Use Modbus from
      | Console
  MainsCon : Inport
  Bus Creator1 : BusCreator  Inputs=2
  Bus Creator12 : BusCreator  Inputs=8
  Fcmd pu : Constant  Value=1.0
  Gain1 : Gain  Gain=2  OutDataTypeStr=double
  Gain2 : Gain
  Gain3 : Gain  Gain=4000
  Gain4 : Gain  Gain=4000
  Gain5 : Gain  Gain=4800
  Gain6 : Gain  Gain=6000
  Gain7 : Gain  Gain=8
  Logical Operator : Logic  Operator=NOT  AllPortsSameDT=off  OutDataTypeStr=boolean
  Manual Switch1 : ManualSwitch  CurrentSetting=0
  Manual Switch2 : ManualSwitch
  Manual Switch3 : ManualSwitch
  Manual Switch4 : ManualSwitch
  PCmd1 : Constant  Value=300
  PCmd2 : Constant  Value=300
  PCmd3 : Constant  Value=0
  PCmd4 : Constant  Value=0
  PCmd5 : Constant  Value=9
  PCmd6 : Constant  Value=0
  PCmd7 : Constant
  PCmd8 : Constant  Value=11
  Pfactor : Gain  Gain=.9
  Qfactor : Gain  Gain=.43
  Rate Transition : RateTransition  Deterministic=off
  Rate Transition1 : RateTransition  Deterministic=off
  S Profile1 : simulink/Sources/Repeating Sequence Stair  OutValues=Stim.Gen3.Ena  tsamp=[Stim.Ts Ts]  OutMin=[]  OutMax=[]  OutDataTypeStr=Inherit: Inherit via back propagation  OutDataType=fixdt(0,8)  ConRadixGroup=Best Precision: Vector-wise  OutScaling=2^-12
  S Profile2 : simulink/Sources/Repeating Sequence Stair  OutValues=Stim.Gen3.Run  tsamp=[Stim.Ts Ts]  OutMin=[]  OutMax=[]  OutDataTypeStr=Inherit: Inherit via back propagation  OutDataType=fixdt(0,8)  ConRadixGroup=Best Precision: Vector-wise  OutScaling=2^-12
  S Profile3 : simulink/Sources/Repeating Sequence Stair  OutValues=Stim.Gen3.s  tsamp=[Stim.Ts Ts]  OutMin=[]  OutMax=[]  OutDataTypeStr=Inherit: Inherit via back propagation  OutDataType=fixdt(0,8)  ConRadixGroup=Best Precision: Vector-wise  OutScaling=2^-12
  Sum : Sum  Inputs=+++
  Vcmd pu : Constant
  MbCtrl : Outport
  wires:
  MainsCon/1 -> Rate Transition1/1
  Logical Operator/1 -> Gain1/1  "VF_control"
  Gain7/1 -> Sum/3
  S Profile2/1 -> Gain7/1  "Run"
  Gain6/1 -> Bus Creator12/5  "FreqCmd"
  Gain5/1 -> Bus Creator12/4  "VoltCmd"
  Gain4/1 -> Bus Creator12/3  "QCmd"
  Gain3/1 -> Bus Creator12/2  "PCmd"
  PCmd7/1 -> Manual Switch4/2
  PCmd6/1 -> Manual Switch4/1
  Manual Switch4/1 -> Bus Creator1/2  "ModbusEnable"
  Bus Creator1/1 -> Rate Transition/1
  PCmd5/1 -> Bus Creator12/8
  PCmd2/1 -> Bus Creator12/7
  PCmd1/1 -> Bus Creator12/6
  Sum/1 -> Manual Switch1/1  "Ctrl"
  Gain1/1 -> Sum/2
  Gain2/1 -> Sum/1
  PCmd3/1 -> Manual Switch2/2
  PCmd4/1 -> Manual Switch3/2
  Manual Switch3/1 -> Gain4/1
  Bus Creator12/1 -> Bus Creator1/1  "ModbusFromSC"
  Manual Switch2/1 -> Gain3/1
  S Profile1/1 -> Gain2/1  "Enable"
  Pfactor/1 -> Manual Switch2/1  "P"
  Fcmd pu/1 -> Gain6/1  "F"
  Vcmd pu/1 -> Gain5/1  "V"
  Qfactor/1 -> Manual Switch3/1  "Q"
  S Profile3/1 -> Qfactor/1, Pfactor/1  "P"
  Rate Transition/1 -> MbCtrl/1
  Rate Transition1/1 -> Logical Operator/1
  PCmd8/1 -> Manual Switch1/2
  Manual Switch1/1 -> Bus Creator12/1  "Ctrl"

== system UrbanCHIL/SC_ctrl/IO_scaling ==
  Bus Creator12 : BusCreator  Inputs=8
  Manual Switch : ManualSwitch
  PCmd1 : Constant
  PCmd2 : Constant  Value=[ 6 6 6 ]
  PCmd3 : Constant
  PCmd4 : Constant  Value=125
  PCmd5 : Constant  Value=6
  PCmd6 : Constant
  PCmd7 : Constant  Value=10/600
  Real_measurements : Constant
  Sim_measurements : Constant  Value=0
  Out1 : Outport
  wires:
  PCmd7/1 -> Bus Creator12/3  "AOUT_I_GAIN"
  Bus Creator12/1 -> Out1/1
  PCmd6/1 -> Bus Creator12/2  "AIN_I_GAIN"
  PCmd3/1 -> Bus Creator12/1  "AIN_V_GAIN"
  PCmd1/1 -> Bus Creator12/4  "AOUT_V_GAIN"
  Manual Switch/1 -> Bus Creator12/5  "PHIL_Enabled"
  Real_measurements/1 -> Manual Switch/2  "record_rms_signals"
  Sim_measurements/1 -> Manual Switch/1
  PCmd4/1 -> Bus Creator12/6  "I_sense_gain"
  PCmd5/1 -> Bus Creator12/7  "I_sense_offset"
  PCmd2/1 -> Bus Creator12/8  "I_gen_offset"

== system UrbanCHIL/SC_ctrl/PV1 control ==
  note: Use Modbus TCP
  note: Use Modbus from
      | Console
  Bus Creator1 : BusCreator  Inputs=3
  Bus Creator12 : BusCreator  Inputs=8
  Gain3 : Gain  Gain=5000
  Gain4 : Gain  Gain=5000
  Gain5 : Gain  Gain=4800
  Gain6 : Gain  Gain=6000
  Manual Switch : ManualSwitch  CurrentSetting=0
  Manual Switch1 : ManualSwitch  CurrentSetting=0
  Manual Switch2 : ManualSwitch
  Manual Switch3 : ManualSwitch  CurrentSetting=0
  PCmd{1..2,4,6} (4 alike) : Constant  Value=0
  PCmd3 : Constant  Value=0.7
  PCmd5 : Constant  Value=11
  PCmd7 : Constant
  PCmd8 : Constant
  Rate Transition : RateTransition  Deterministic=off
  S Profile1 : simulink/Sources/Repeating Sequence Stair  OutValues=Stim.PV2.Ena  tsamp=[Stim.Ts Ts]  OutMin=[]  OutMax=[]  OutDataTypeStr=Inherit: Inherit via back propagation  OutDataType=fixdt(0,8)  ConRadixGroup=Best Precision: Vector-wise  OutScaling=2^-12
  S Profile2 : simulink/Sources/Repeating Sequence Stair  OutValues=Stim.ESS2.p  tsamp=[Stim.Ts Ts]  OutMin=[]  OutMax=[]  OutDataTypeStr=Inherit: Inherit via back propagation  OutDataType=fixdt(0,8)  ConRadixGroup=Best Precision: Vector-wise  OutScaling=2^-12
  S Profile3 : simulink/Sources/Repeating Sequence Stair  OutValues=Stim.ESS2.q  tsamp=[Stim.Ts Ts]  OutMin=[]  OutMax=[]  OutDataTypeStr=Inherit: Inherit via back propagation  OutDataType=fixdt(0,8)  ConRadixGroup=Best Precision: Vector-wise  OutScaling=2^-12
  S Profile4 : simulink/Sources/Repeating Sequence Stair  OutValues=Stim.ESS2.v  tsamp=[Stim.Ts Ts]  OutMin=[]  OutMax=[]  OutDataTypeStr=Inherit: Inherit via back propagation  OutDataType=fixdt(0,8)  ConRadixGroup=Best Precision: Vector-wise  OutScaling=2^-12
  S Profile5 : simulink/Sources/Repeating Sequence Stair  OutValues=Stim.ESS2.f  tsamp=[Stim.Ts Ts]  OutMin=[]  OutMax=[]  OutDataTypeStr=Inherit: Inherit via back propagation  OutDataType=fixdt(0,8)  ConRadixGroup=Best Precision: Vector-wise  OutScaling=2^-12
  Tuning : Subsystem
  Out1 : Outport
  wires:
  Rate Transition/1 -> Out1/1
  Gain6/1 -> Bus Creator12/5  "FreqCmd"
  Gain5/1 -> Bus Creator12/4  "VoltCmd"
  Gain4/1 -> Bus Creator12/3  "QCmd"
  Gain3/1 -> Bus Creator12/2  "PCmd"
  PCmd7/1 -> Manual Switch2/2
  PCmd6/1 -> Manual Switch2/1
  Manual Switch2/1 -> Bus Creator1/2  "ModbusEnable"
  Bus Creator1/1 -> Rate Transition/1
  PCmd5/1 -> Bus Creator12/8
  PCmd2/1 -> Bus Creator12/7
  PCmd1/1 -> Bus Creator12/6
  S Profile1/1 -> Manual Switch3/1
  S Profile3/1 -> Manual Switch1/1
  S Profile2/1 -> Manual Switch/1
  PCmd3/1 -> Manual Switch/2
  PCmd4/1 -> Manual Switch1/2
  S Profile4/1 -> Gain5/1
  Manual Switch1/1 -> Gain4/1
  Bus Creator12/1 -> Bus Creator1/1  "ModbusFromSC"
  Manual Switch/1 -> Gain3/1
  S Profile5/1 -> Gain6/1
  PCmd8/1 -> Manual Switch3/2
  Manual Switch3/1 -> Bus Creator12/1  "Ctrl"
  Tuning/1(Tuning) -> Bus Creator1/3  "Tuning"
